simulink model "rdc_bl"  (Simulink 8.1)
settings: Solver=ode45  StartTime=0.0  StopTime=10.0  RelTol=1e-3
undefined symbols (not defined in the file or in its folder): R_BL, Rco, Rd, Rpt, Rr, Rs, Rt
settings Model: Creator=kartik.karuna  LastModifiedBy=kartik.karuna
settings DataIOCC: SignalLoggingSaveFormat=Dataset
settings OptimizationCC: ExpressionDepthLimit=128
settings DebuggingCC: FcnCallInpInsideContextMsg=EnableAllAsError
settings GRTTargetCC: CombineOutputUpdateFcns=on  GRTInterface=off

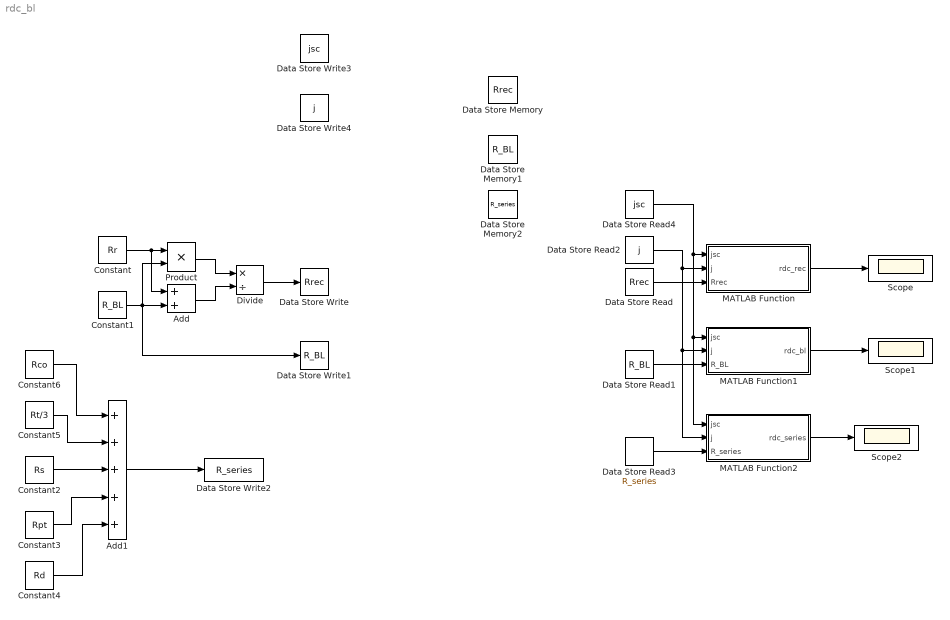
== system rdc_bl ==
  Add : Sum
  Add1 : Sum  Inputs=+++++
  Constant : Constant  Value=Rr
  Constant1 : Constant  Value=R_BL
  Constant2 : Constant  Value=Rs
  Constant3 : Constant  Value=Rpt
  Constant4 : Constant  Value=Rd
  Constant5 : Constant  Value=Rt/3
  Constant6 : Constant  Value=Rco
  Data Store Memory : DataStoreMemory  DataStoreName=Rrec  ReadBeforeWriteMsg=warning  WriteAfterWriteMsg=warning  WriteAfterReadMsg=warning
  Data Store Memory1 : DataStoreMemory  DataStoreName=R_BL  ReadBeforeWriteMsg=warning  WriteAfterWriteMsg=warning  WriteAfterReadMsg=warning
  Data Store Memory2 : DataStoreMemory  DataStoreName=R_series  ReadBeforeWriteMsg=warning  WriteAfterWriteMsg=warning  WriteAfterReadMsg=warning
  Data Store Read : DataStoreRead  DataStoreName=Rrec
  Data Store Read1 : DataStoreRead  DataStoreName=R_BL
  Data Store Read2 : DataStoreRead  DataStoreName=j
  Data Store Read3 : DataStoreRead  DataStoreName=R_series
  Data Store Read4 : DataStoreRead  DataStoreName=jsc
  Data Store Write : DataStoreWrite  DataStoreName=Rrec
  Data Store Write1 : DataStoreWrite  DataStoreName=R_BL
  Data Store Write2 : DataStoreWrite  DataStoreName=R_series
  Data Store Write3 : DataStoreWrite  DataStoreName=jsc
  Data Store Write4 : DataStoreWrite  DataStoreName=j
  Divide : Product  Inputs=*/
  MATLAB Function : MATLAB Function  TreatAsAtomicUnit=on
  MATLAB Function1 : MATLAB Function  TreatAsAtomicUnit=on
  MATLAB Function2 : MATLAB Function  TreatAsAtomicUnit=on
  Product : Product
  Scope : Scope
  Scope1 : Scope
  Scope2 : Scope
      settings: SaveName=ScopeData2
  wires:
  Data Store Read/1 -> MATLAB Function/3(Rrec)
  Data Store Read1/1 -> MATLAB Function1/3(R_BL)
  Data Store Read3/1 -> MATLAB Function2/3(R_series)
  Data Store Read2/1 -> MATLAB Function2/2(j), MATLAB Function1/2(j), MATLAB Function/2(j)
  Data Store Read4/1 -> MATLAB Function2/1(jsc), MATLAB Function1/1(jsc), MATLAB Function/1(jsc)
  MATLAB Function/1(rdc_rec) -> Scope/1
  MATLAB Function1/1(rdc_bl) -> Scope1/1
  MATLAB Function2/1(rdc_series) -> Scope2/1
  Constant/1 -> Add/1, Product/1
  Constant1/1 -> Product/2, Data Store Write1/1, Add/2
  Product/1 -> Divide/1
  Add/1 -> Divide/2
  Divide/1 -> Data Store Write/1
  Constant3/1 -> Add1/4
  Constant4/1 -> Add1/5
  Constant2/1 -> Add1/3
  Constant5/1 -> Add1/2
  Constant6/1 -> Add1/1
  Add1/1 -> Data Store Write2/1

== matlab function MATLAB Function1 ==
  data: jsc input double; rdc_bl output double; j input double; R_BL input double
function rdc_bl = f_rdcbl(jsc,j,R_BL)
%#codegen

rdc_bl = 1/(jsc-j)*integral(R_BL,jsc,j);

== matlab function MATLAB Function ==
  data: jsc input double; rdc_rec output double; j input double; Rrec input double
function rdc_rec = f_rdcrec(jsc,j,Rrec)
%#codegen

rdc_rec = 1/(jsc-j)*integral(Rrec,jsc,j);

== matlab function MATLAB Function2 ==
  data: jsc input double; rdc_series output double; j input double; R_series input double
function rdc_series = f_rdser(jsc,j,R_series)
%#codegen

rdc_series = 1/(jsc-j)*integral(R_series,jsc,j);
